simulink subsystem "Mq_SubSystem"  (R2020b)
settings: Solver=VariableStepAuto  StartTime=0.0  StopTime=10.0  RelTol=1e-3
undefined symbols (not defined in the file or in its folder): Irotyy, l, M11q, M22q, mb, mrot, n, r, Ts, zbrot
settings Model: Creator=umberto  LastModifiedBy=umberto

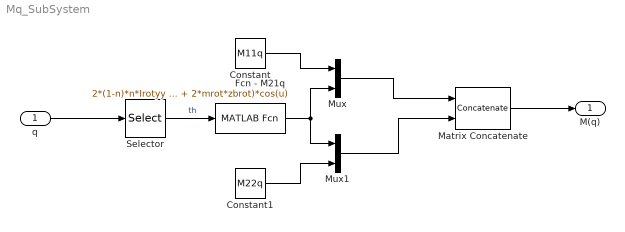
== system Mq_SubSystem ==
  q : Inport
  Constant : Constant  Value=M11q  SampleTime=Ts
  Constant1 : Constant  Value=M22q  SampleTime=Ts
  Fcn - M21q : MATLABFcn  MATLABFcn=2*(1-n)*n*Irotyy + r*(l*mb + 2*mrot*zbrot)*cos(u)
  Matrix Concatenate : Concatenate  Mode=Multidimensional array  ConcatenateDimension=2
  Mux : Mux  Inputs=2
  Mux1 : Mux  Inputs=2
  Selector : Selector  InputPortWidth=2  IndexOptions=Index vector (dialog)  Indices=[2]  OutputSizes=1
  M(q) : Outport
  wires:
  q/1 -> Selector/1
  Selector/1 -> Fcn - M21q/1  "th"
  Fcn - M21q/1 -> Mux/2, Mux1/1
  Constant1/1 -> Mux1/2
  Constant/1 -> Mux/1
  Mux/1 -> Matrix Concatenate/1
  Mux1/1 -> Matrix Concatenate/2
  Matrix Concatenate/1 -> M(q)/1
